simulink model "PIDControllerTest"  (R2025b)
settings: Solver=FixedStepAuto  StartTime=0.0  StopTime=inf  FixedStep=.01  RelTol=1e-3
settings Model: Creator=talles  LastModifiedBy=ajax

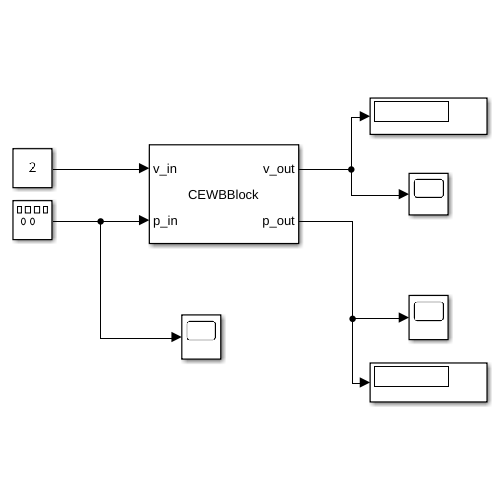
[thumbnail: Simulink's stored preview of the top-level diagram]
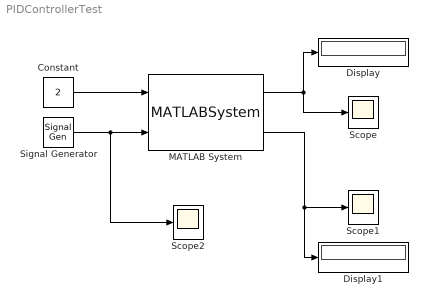
== system PIDControllerTest ==
  Constant : Constant  Value=2
  Display : Display
  Display1 : Display
  MATLAB System : MATLABSystem  System=CEWBBlock  COMPort=/dev/ttyACM0  BaudRate=115200  SimulateUsing=Code generation
      mask Type: CEWBBlock
  Scope : Scope
      settings: ActiveDisplayYMinimum=1  ActiveDisplayYMaximum=3
  Scope1 : Scope
      settings: ActiveDisplayYMinimum=-6.0034594760493682  ActiveDisplayYMaximum=14.706273819701902
  Scope2 : Scope
      settings: ActiveDisplayYMinimum=-0.98168540283123717  ActiveDisplayYMaximum=1.0032543199733903  DataLoggingVariableName=ScopeData2
  Signal Generator : SignalGenerator  Amplitude=1000
  wires:
  MATLAB System/1 -> Scope/1, Display/1
  MATLAB System/2 -> Display1/1, Scope1/1
  Signal Generator/1 -> Scope2/1, MATLAB System/2
  Constant/1 -> MATLAB System/1
